simulink model "stereo_ibvs_ros_backup_20260724_144900"  (R2025b)
settings: Solver=FixedStepDiscrete  StartTime=0.0  StopTime=inf  FixedStep=cfg.Ts  RelTol=1e-3
InitFcn:
  | modelPath = get_param(bdroot,'FileName');
  |                                                                                       simulinkPath = fileparts(fileparts(modelPath));
  |                                                                                       projectRoot = fileparts(simulinkPath);
  |                                                                                       configPath = fullfile(simulinkPath,'config','stereo_ibvs_config.m');
  |                                                                                       corePath = fullfile(simulinkPath,'core');
  |                                                                                       generatedPath = fullfile(projectRoot,'matlab_msg_gen',computer('arch'),'install','m');
  |                                                                                       if ~isfile(configPath), error('StereoIBVS:ConfigNotFound','找不到配置文件：%s',configPath); end
  |                                                                                       addpath(corePath);
  |                                                                                       if isfolder(generatedPath), addpath(generatedPath,'-begin'); end
  |                                                                                       run(configPath);
undefined symbols (not defined in the file): cfg, data, data_SL_Info
libraries: ros2lib x10
settings Model: Creator=hlc  LastModifiedBy=hlc
settings DataIOCC: SaveOutput=off  SaveTime=off  ReturnWorkspaceOutputs=off

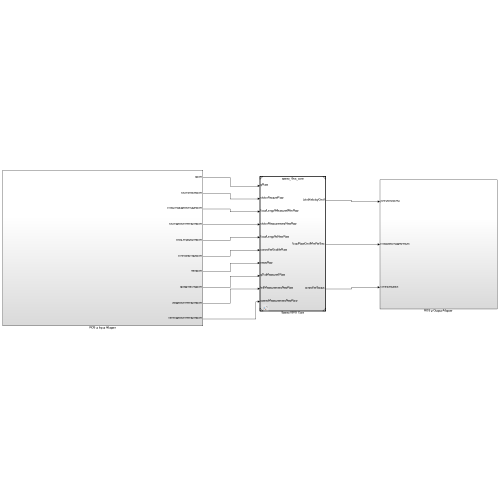
[thumbnail: Simulink's stored preview of the top-level diagram]
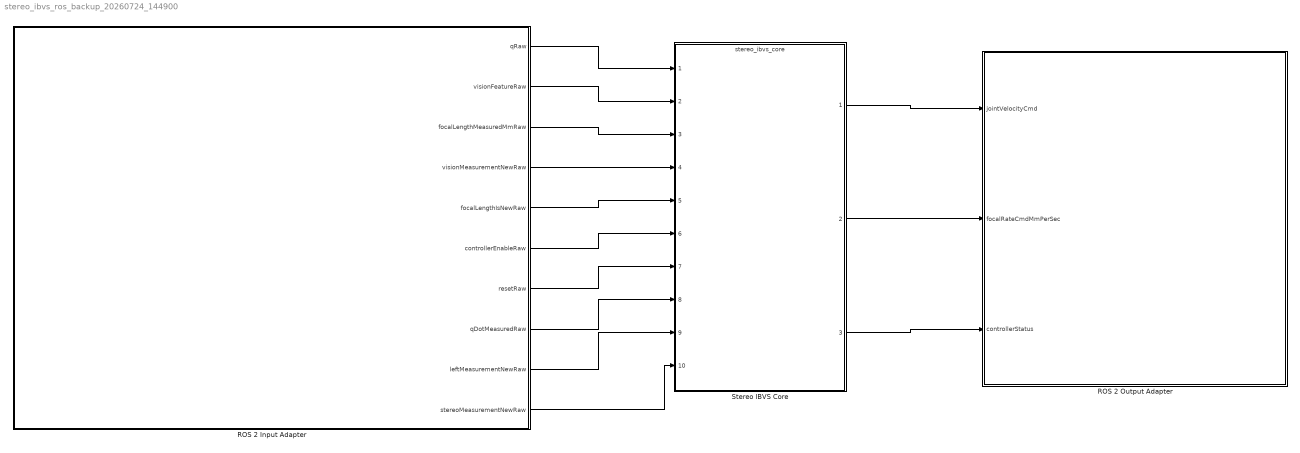
== system stereo_ibvs_ros_backup_20260724_144900 ==
  ROS 2 Input Adapter : Subsystem
  ROS 2 Output Adapter : Subsystem
  Stereo IBVS Core : ModelReference  ModelNameDialog=stereo_ibvs_core  SimulationMode=Normal  ModelReferenceVersion=1.1
  wires:
  ROS 2 Input Adapter/1(qRaw) -> Stereo IBVS Core/1
  ROS 2 Input Adapter/2(visionFeatureRaw) -> Stereo IBVS Core/2
  ROS 2 Input Adapter/3(focalLengthMeasuredMmRaw) -> Stereo IBVS Core/3
  ROS 2 Input Adapter/4(visionMeasurementNewRaw) -> Stereo IBVS Core/4
  ROS 2 Input Adapter/5(focalLengthIsNewRaw) -> Stereo IBVS Core/5
  ROS 2 Input Adapter/6(controllerEnableRaw) -> Stereo IBVS Core/6
  ROS 2 Input Adapter/7(resetRaw) -> Stereo IBVS Core/7
  ROS 2 Input Adapter/8(qDotMeasuredRaw) -> Stereo IBVS Core/8
  ROS 2 Input Adapter/9(leftMeasurementNewRaw) -> Stereo IBVS Core/9
  ROS 2 Input Adapter/10(stereoMeasurementNewRaw) -> Stereo IBVS Core/10
  Stereo IBVS Core/1 -> ROS 2 Output Adapter/1(jointVelocityCmd)
  Stereo IBVS Core/2 -> ROS 2 Output Adapter/2(focalRateCmdMmPerSec)
  Stereo IBVS Core/3 -> ROS 2 Output Adapter/3(controllerStatus)

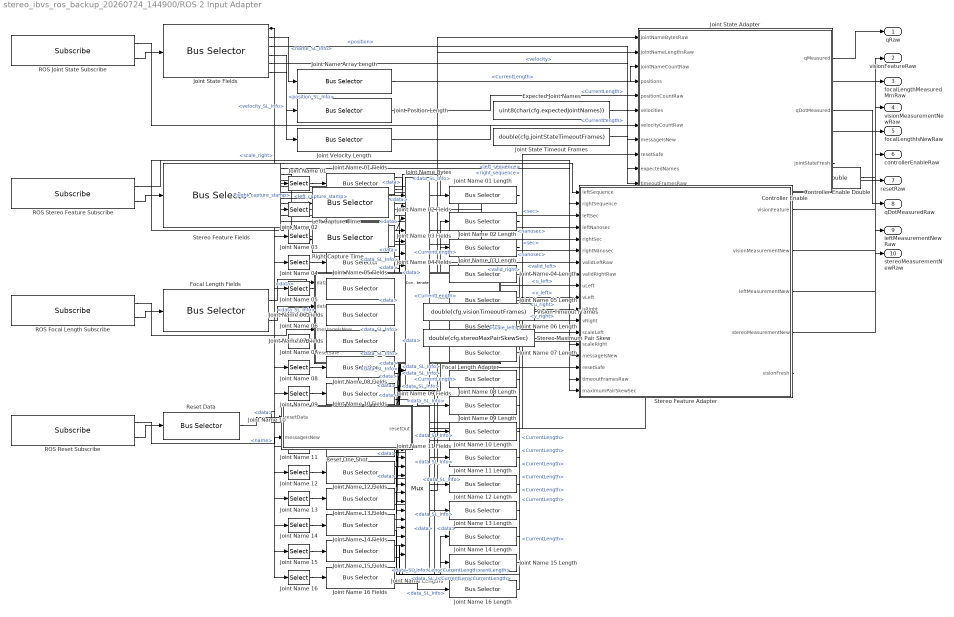
== system stereo_ibvs_ros_backup_20260724_144900/ROS 2 Input Adapter ==
  Controller Enable : Logic  AllPortsSameDT=off  OutDataTypeStr=boolean
  Controller Enable Double : DataTypeConversion  OutDataTypeStr=double  SaturateOnIntegerOverflow=off  RndMeth=Floor
  Expected Joint Names : Constant  Value=uint8(char(cfg.expectedJointNames))  SampleTime=-1
  Focal Length Adapter : MATLAB Function  TreatAsAtomicUnit=on
  Focal Length Fields : BusSelector  OutputSignals=data,data_SL_Info
  Joint Name 01 : Selector  InputPortWidth=16  IndexOptions=Index vector (dialog)  Indices=1  OutputSizes=1
  Joint Name 01 Fields : BusSelector  OutputSignals=data,data_SL_Info
  Joint Name 01 Length : BusSelector  OutputSignals=CurrentLength
  Joint Name 02 : Selector  InputPortWidth=16  IndexOptions=Index vector (dialog)  Indices=2  OutputSizes=1
  Joint Name 02 Fields : BusSelector  OutputSignals=data,data_SL_Info
  Joint Name 02 Length : BusSelector  OutputSignals=CurrentLength
  Joint Name 03 : Selector  InputPortWidth=16  IndexOptions=Index vector (dialog)  Indices=3  OutputSizes=1
  Joint Name 03 Fields : BusSelector  OutputSignals=data,data_SL_Info
  Joint Name 03 Length : BusSelector  OutputSignals=CurrentLength
  Joint Name 04 : Selector  InputPortWidth=16  IndexOptions=Index vector (dialog)  Indices=4  OutputSizes=1
  Joint Name 04 Fields : BusSelector  OutputSignals=data,data_SL_Info
  Joint Name 04 Length : BusSelector  OutputSignals=CurrentLength
  Joint Name 05 : Selector  InputPortWidth=16  IndexOptions=Index vector (dialog)  Indices=5  OutputSizes=1
  Joint Name 05 Fields : BusSelector  OutputSignals=data,data_SL_Info
  Joint Name 05 Length : BusSelector  OutputSignals=CurrentLength
  Joint Name 06 : Selector  InputPortWidth=16  IndexOptions=Index vector (dialog)  Indices=6  OutputSizes=1
  Joint Name 06 Fields : BusSelector  OutputSignals=data,data_SL_Info
  Joint Name 06 Length : BusSelector  OutputSignals=CurrentLength
  Joint Name 07 : Selector  InputPortWidth=16  IndexOptions=Index vector (dialog)  Indices=7  OutputSizes=1
  Joint Name 07 Fields : BusSelector  OutputSignals=data,data_SL_Info
  Joint Name 07 Length : BusSelector  OutputSignals=CurrentLength
  Joint Name 08 : Selector  InputPortWidth=16  IndexOptions=Index vector (dialog)  Indices=8  OutputSizes=1
  Joint Name 08 Fields : BusSelector  OutputSignals=data,data_SL_Info
  Joint Name 08 Length : BusSelector  OutputSignals=CurrentLength
  Joint Name 09 : Selector  InputPortWidth=16  IndexOptions=Index vector (dialog)  Indices=9  OutputSizes=1
  Joint Name 09 Fields : BusSelector  OutputSignals=data,data_SL_Info
  Joint Name 09 Length : BusSelector  OutputSignals=CurrentLength
  Joint Name 10 : Selector  InputPortWidth=16  IndexOptions=Index vector (dialog)  Indices=10  OutputSizes=1
  Joint Name 10 Fields : BusSelector  OutputSignals=data,data_SL_Info
  Joint Name 10 Length : BusSelector  OutputSignals=CurrentLength
  Joint Name 11 : Selector  InputPortWidth=16  IndexOptions=Index vector (dialog)  Indices=11  OutputSizes=1
  Joint Name 11 Fields : BusSelector  OutputSignals=data,data_SL_Info
  Joint Name 11 Length : BusSelector  OutputSignals=CurrentLength
  Joint Name 12 : Selector  InputPortWidth=16  IndexOptions=Index vector (dialog)  Indices=12  OutputSizes=1
  Joint Name 12 Fields : BusSelector  OutputSignals=data,data_SL_Info
  Joint Name 12 Length : BusSelector  OutputSignals=CurrentLength
  Joint Name 13 : Selector  InputPortWidth=16  IndexOptions=Index vector (dialog)  Indices=13  OutputSizes=1
  Joint Name 13 Fields : BusSelector  OutputSignals=data,data_SL_Info
  Joint Name 13 Length : BusSelector  OutputSignals=CurrentLength
  Joint Name 14 : Selector  InputPortWidth=16  IndexOptions=Index vector (dialog)  Indices=14  OutputSizes=1
  Joint Name 14 Fields : BusSelector  OutputSignals=data,data_SL_Info
  Joint Name 14 Length : BusSelector  OutputSignals=CurrentLength
  Joint Name 15 : Selector  InputPortWidth=16  IndexOptions=Index vector (dialog)  Indices=15  OutputSizes=1
  Joint Name 15 Fields : BusSelector  OutputSignals=data,data_SL_Info
  Joint Name 15 Length : BusSelector  OutputSignals=CurrentLength
  Joint Name 16 : Selector  InputPortWidth=16  IndexOptions=Index vector (dialog)  Indices=16  OutputSizes=1
  Joint Name 16 Fields : BusSelector  OutputSignals=data,data_SL_Info
  Joint Name 16 Length : BusSelector  OutputSignals=CurrentLength
  Joint Name Array Length : BusSelector  OutputSignals=CurrentLength
  Joint Name Bytes : Concatenate  NumInputs=16
  Joint Name Lengths : Mux  Inputs=16
  Joint Position Length : BusSelector  OutputSignals=CurrentLength
  Joint State Adapter : MATLAB Function  TreatAsAtomicUnit=on
  Joint State Fields : BusSelector  OutputSignals=name,name_SL_Info,position,position_SL_Info,velocity,velocity_SL_Info
  Joint State Timeout Frames : Constant  Value=double(cfg.jointStateTimeoutFrames)  OutDataTypeStr=double  SampleTime=-1
  Joint Velocity Length : BusSelector  OutputSignals=CurrentLength
  Left Capture Time : BusSelector  OutputSignals=sec,nanosec
  ROS Focal Length Subscribe : ros2lib/Subscribe  topicSource=Specify your own  topic=/stereo/focal_length  messageType=std_msgs/Float64MultiArray  sampleTime=cfg.Ts  QOSHistory=Keep last  QOSDepth=10  QOSReliability=Reliable  QOSDurability=Volatile  QOSDeadline=Inf  QOSLifespan=Inf  QOSLiveliness=Automatic  QOSLeaseDuration=Inf  QOSAvoidROSNamespaceConventions=off
  ROS Joint State Subscribe : ros2lib/Subscribe  topicSource=Specify your own  topic=/franka/joint_states  messageType=sensor_msgs/JointState  sampleTime=cfg.Ts  QOSHistory=Keep last  QOSDepth=10  QOSReliability=Reliable  QOSDurability=Volatile  QOSDeadline=Inf  QOSLifespan=Inf  QOSLiveliness=Automatic  QOSLeaseDuration=Inf  QOSAvoidROSNamespaceConventions=off
  ROS Reset Subscribe : ros2lib/Subscribe  topicSource=Specify your own  topic=/simulink/reset  messageType=std_msgs/Bool  sampleTime=cfg.Ts  QOSHistory=Keep last  QOSDepth=10  QOSReliability=Reliable  QOSDurability=Volatile  QOSDeadline=Inf  QOSLifespan=Inf  QOSLiveliness=Automatic  QOSLeaseDuration=Inf  QOSAvoidROSNamespaceConventions=off
  ROS Stereo Feature Subscribe : ros2lib/Subscribe  topicSource=Specify your own  topic=/vision_double/stereo_features  messageType=velocity_servo_tag_interfaces/StereoFeatures  sampleTime=cfg.Ts  QOSHistory=Keep last  QOSDepth=10  QOSReliability=Reliable  QOSDurability=Volatile  QOSDeadline=Inf  QOSLifespan=Inf  QOSLiveliness=Automatic  QOSLeaseDuration=Inf  QOSAvoidROSNamespaceConventions=off
  Reset Data : BusSelector  OutputSignals=data
  Reset One Shot : MATLAB Function  TreatAsAtomicUnit=on
  Right Capture Time : BusSelector  OutputSignals=sec,nanosec
  Stereo Feature Adapter : MATLAB Function  TreatAsAtomicUnit=on
  Stereo Feature Fields : BusSelector  OutputSignals=left_sequence,right_sequence,left_capture_stamp,right_capture_stamp,valid_left,valid_right,u_left,v_left,u_right,v_right,scale_left,scale_right
  Stereo Maximum Pair Skew : Constant  Value=double(cfg.stereoMaxPairSkewSec)  OutDataTypeStr=double  SampleTime=-1
  Vision Timeout Frames : Constant  Value=double(cfg.visionTimeoutFrames)  OutDataTypeStr=double  SampleTime=-1
  qRaw : Outport  PortDimensions=[7 1]
  visionFeatureRaw : Outport  Port=2  PortDimensions=[8 1]
  focalLengthMeasuredMmRaw : Outport  Port=3  PortDimensions=[2 1]
  visionMeasurementNewRaw : Outport  Port=4  PortDimensions=1
  focalLengthIsNewRaw : Outport  Port=5  PortDimensions=1
  controllerEnableRaw : Outport  Port=6  PortDimensions=1
  resetRaw : Outport  Port=7  PortDimensions=1
  qDotMeasuredRaw : Outport  Port=8  PortDimensions=[7 1]
  leftMeasurementNewRaw : Outport  Port=9  PortDimensions=1
  stereoMeasurementNewRaw : Outport  Port=10  PortDimensions=1
  wires:
  ? -> ?
  ROS Reset Subscribe/2 -> Reset Data/1
  Reset Data/1 -> Reset One Shot/1(resetData)  "<data>"
  ROS Reset Subscribe/1 -> Reset One Shot/2(messageIsNew)
  Joint State Fields/1 -> Joint Name 01/1, Joint Name 02/1, Joint Name 03/1, Joint Name 04/1, Joint Name 05/1, Joint Name 06/1, Joint Name 07/1, Joint Name 08/1, Joint Name 09/1, Joint Name 10/1, Joint Name 11/1, Joint Name 12/1, Joint Name 13/1, Joint Name 14/1, Joint Name 15/1, Joint Name 16/1  "<name>"
  Joint Name 01/1 -> Joint Name 01 Fields/1
  Joint Name 01 Fields/1 -> Joint Name Bytes/1  "<data>"
  Joint Name 01 Fields/2 -> Joint Name 01 Length/1  "<data_SL_Info>"
  Joint Name 01 Length/1 -> Joint Name Lengths/1  "<CurrentLength>"
  Joint Name 02/1 -> Joint Name 02 Fields/1
  Joint Name 02 Fields/1 -> Joint Name Bytes/2  "<data>"
  Joint Name 02 Fields/2 -> Joint Name 02 Length/1  "<data_SL_Info>"
  Joint Name 02 Length/1 -> Joint Name Lengths/2  "<CurrentLength>"
  Joint Name 03/1 -> Joint Name 03 Fields/1
  Joint Name 03 Fields/1 -> Joint Name Bytes/3  "<data>"
  Joint Name 03 Fields/2 -> Joint Name 03 Length/1  "<data_SL_Info>"
  Joint Name 03 Length/1 -> Joint Name Lengths/3  "<CurrentLength>"
  Joint Name 04/1 -> Joint Name 04 Fields/1
  Joint Name 04 Fields/1 -> Joint Name Bytes/4  "<data>"
  Joint Name 04 Fields/2 -> Joint Name 04 Length/1  "<data_SL_Info>"
  Joint Name 04 Length/1 -> Joint Name Lengths/4  "<CurrentLength>"
  Joint Name 05/1 -> Joint Name 05 Fields/1
  Joint Name 05 Fields/1 -> Joint Name Bytes/5  "<data>"
  Joint Name 05 Fields/2 -> Joint Name 05 Length/1  "<data_SL_Info>"
  Joint Name 05 Length/1 -> Joint Name Lengths/5  "<CurrentLength>"
  Joint Name 06/1 -> Joint Name 06 Fields/1
  Joint Name 06 Fields/1 -> Joint Name Bytes/6  "<data>"
  Joint Name 06 Fields/2 -> Joint Name 06 Length/1  "<data_SL_Info>"
  Joint Name 06 Length/1 -> Joint Name Lengths/6  "<CurrentLength>"
  Joint Name 07/1 -> Joint Name 07 Fields/1
  Joint Name 07 Fields/1 -> Joint Name Bytes/7  "<data>"
  Joint Name 07 Fields/2 -> Joint Name 07 Length/1  "<data_SL_Info>"
  Joint Name 07 Length/1 -> Joint Name Lengths/7  "<CurrentLength>"
  Joint Name 08/1 -> Joint Name 08 Fields/1
  Joint Name 08 Fields/1 -> Joint Name Bytes/8  "<data>"
  Joint Name 08 Fields/2 -> Joint Name 08 Length/1  "<data_SL_Info>"
  Joint Name 08 Length/1 -> Joint Name Lengths/8  "<CurrentLength>"
  Joint Name 09/1 -> Joint Name 09 Fields/1
  Joint Name 09 Fields/1 -> Joint Name Bytes/9  "<data>"
  Joint Name 09 Fields/2 -> Joint Name 09 Length/1  "<data_SL_Info>"
  Joint Name 09 Length/1 -> Joint Name Lengths/9  "<CurrentLength>"
  Joint Name 10/1 -> Joint Name 10 Fields/1
  Joint Name 10 Fields/1 -> Joint Name Bytes/10  "<data>"
  Joint Name 10 Fields/2 -> Joint Name 10 Length/1  "<data_SL_Info>"
  Joint Name 10 Length/1 -> Joint Name Lengths/10  "<CurrentLength>"
  Joint Name 11/1 -> Joint Name 11 Fields/1
  Joint Name 11 Fields/1 -> Joint Name Bytes/11  "<data>"
  Joint Name 11 Fields/2 -> Joint Name 11 Length/1  "<data_SL_Info>"
  Joint Name 11 Length/1 -> Joint Name Lengths/11  "<CurrentLength>"
  Joint Name 12/1 -> Joint Name 12 Fields/1
  Joint Name 12 Fields/1 -> Joint Name Bytes/12  "<data>"
  Joint Name 12 Fields/2 -> Joint Name 12 Length/1  "<data_SL_Info>"
  Joint Name 12 Length/1 -> Joint Name Lengths/12  "<CurrentLength>"
  Joint Name 13/1 -> Joint Name 13 Fields/1
  Joint Name 13 Fields/1 -> Joint Name Bytes/13  "<data>"
  Joint Name 13 Fields/2 -> Joint Name 13 Length/1  "<data_SL_Info>"
  Joint Name 13 Length/1 -> Joint Name Lengths/13  "<CurrentLength>"
  Joint Name 14/1 -> Joint Name 14 Fields/1
  Joint Name 14 Fields/1 -> Joint Name Bytes/14  "<data>"
  Joint Name 14 Fields/2 -> Joint Name 14 Length/1  "<data_SL_Info>"
  Joint Name 14 Length/1 -> Joint Name Lengths/14  "<CurrentLength>"
  Joint Name 15/1 -> Joint Name 15 Fields/1
  Joint Name 15 Fields/1 -> Joint Name Bytes/15  "<data>"
  Joint Name 15 Fields/2 -> Joint Name 15 Length/1  "<data_SL_Info>"
  Joint Name 15 Length/1 -> Joint Name Lengths/15  "<CurrentLength>"
  Joint Name 16/1 -> Joint Name 16 Fields/1
  Joint Name 16 Fields/1 -> Joint Name Bytes/16  "<data>"
  Joint Name 16 Fields/2 -> Joint Name 16 Length/1  "<data_SL_Info>"
  Joint Name 16 Length/1 -> Joint Name Lengths/16  "<CurrentLength>"
  ROS Joint State Subscribe/2 -> Joint State Fields/1
  Joint State Fields/2 -> Joint Name Array Length/1  "<name_SL_Info>"
  Joint State Fields/4 -> Joint Position Length/1  "<position_SL_Info>"
  Joint State Fields/6 -> Joint Velocity Length/1  "<velocity_SL_Info>"
  Joint Name Bytes/1 -> Joint State Adapter/1(jointNameBytesRaw)
  Joint Name Lengths/1 -> Joint State Adapter/2(jointNameLengthsRaw)
  Joint Name Array Length/1 -> Joint State Adapter/3(jointNameCountRaw)  "<CurrentLength>"
  Joint State Fields/3 -> Joint State Adapter/4(positions)  "<position>"
  Joint Position Length/1 -> Joint State Adapter/5(positionCountRaw)  "<CurrentLength>"
  Joint State Fields/5 -> Joint State Adapter/6(velocities)  "<velocity>"
  Joint Velocity Length/1 -> Joint State Adapter/7(velocityCountRaw)  "<CurrentLength>"
  ROS Joint State Subscribe/1 -> Joint State Adapter/8(messageIsNew)
  Reset One Shot/1(resetOut) -> Joint State Adapter/9(resetSafe), Stereo Feature Adapter/16(resetSafe), Focal Length Adapter/4(resetSafe), resetRaw/1
  Expected Joint Names/1 -> Joint State Adapter/10(expectedNames)
  Joint State Timeout Frames/1 -> Joint State Adapter/11(timeoutFramesRaw)
  ROS Stereo Feature Subscribe/2 -> Stereo Feature Fields/1
  Stereo Feature Fields/3 -> Left Capture Time/1  "<left_capture_stamp>"
  Stereo Feature Fields/4 -> Right Capture Time/1  "<right_capture_stamp>"
  Stereo Feature Fields/1 -> Stereo Feature Adapter/1(leftSequence)  "<left_sequence>"
  Stereo Feature Fields/2 -> Stereo Feature Adapter/2(rightSequence)  "<right_sequence>"
  Left Capture Time/1 -> Stereo Feature Adapter/3(leftSec)  "<sec>"
  Left Capture Time/2 -> Stereo Feature Adapter/4(leftNanosec)  "<nanosec>"
  Right Capture Time/1 -> Stereo Feature Adapter/5(rightSec)  "<sec>"
  Right Capture Time/2 -> Stereo Feature Adapter/6(rightNanosec)  "<nanosec>"
  Stereo Feature Fields/5 -> Stereo Feature Adapter/7(validLeftRaw)  "<valid_left>"
  Stereo Feature Fields/6 -> Stereo Feature Adapter/8(validRightRaw)  "<valid_right>"
  Stereo Feature Fields/7 -> Stereo Feature Adapter/9(uLeft)  "<u_left>"
  Stereo Feature Fields/8 -> Stereo Feature Adapter/10(vLeft)  "<v_left>"
  Stereo Feature Fields/9 -> Stereo Feature Adapter/11(uRight)  "<u_right>"
  Stereo Feature Fields/10 -> Stereo Feature Adapter/12(vRight)  "<v_right>"
  Stereo Feature Fields/11 -> Stereo Feature Adapter/13(scaleLeft)  "<scale_left>"
  Stereo Feature Fields/12 -> Stereo Feature Adapter/14(scaleRight)  "<scale_right>"
  ROS Stereo Feature Subscribe/1 -> Stereo Feature Adapter/15(messageIsNew)
  Vision Timeout Frames/1 -> Stereo Feature Adapter/17(timeoutFramesRaw)
  Stereo Maximum Pair Skew/1 -> Stereo Feature Adapter/18(maximumPairSkewSec)
  ROS Focal Length Subscribe/2 -> Focal Length Fields/1
  Focal Length Fields/1 -> Focal Length Adapter/1(data)  "<data>"
  Focal Length Fields/2 -> Focal Length Adapter/2(dataInfo)  "<data_SL_Info>"
  ROS Focal Length Subscribe/1 -> Focal Length Adapter/3(messageIsNew)
  Joint State Adapter/3(jointStateFresh) -> Controller Enable/1
  Stereo Feature Adapter/5(visionFresh) -> Controller Enable/2
  Controller Enable/1 -> Controller Enable Double/1
  Joint State Adapter/1(qMeasured) -> qRaw/1
  Stereo Feature Adapter/1(visionFeature) -> visionFeatureRaw/1
  Focal Length Adapter/1(focalLengthMeasuredMm) -> focalLengthMeasuredMmRaw/1
  Stereo Feature Adapter/2(visionMeasurementNew) -> visionMeasurementNewRaw/1
  Focal Length Adapter/2(focalLengthIsNew) -> focalLengthIsNewRaw/1
  Controller Enable Double/1 -> controllerEnableRaw/1
  Joint State Adapter/2(qDotMeasured) -> qDotMeasuredRaw/1
  Stereo Feature Adapter/3(leftMeasurementNew) -> leftMeasurementNewRaw/1
  Stereo Feature Adapter/4(stereoMeasurementNew) -> stereoMeasurementNewRaw/1

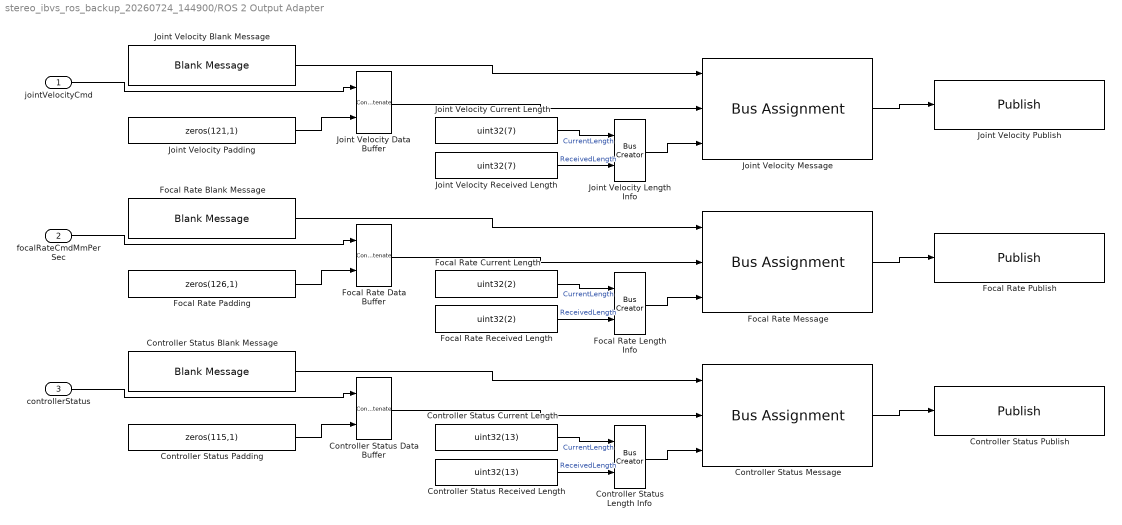
== system stereo_ibvs_ros_backup_20260724_144900/ROS 2 Output Adapter ==
  jointVelocityCmd : Inport  PortDimensions=[7 1]
  focalRateCmdMmPerSec : Inport  Port=2  PortDimensions=[2 1]
  controllerStatus : Inport  Port=3  PortDimensions=[13 1]
  Controller Status Blank Message : ros2lib/Blank Message  messageClass=Message  entityType=std_msgs/Float64MultiArray  messageType=std_msgs/Float64MultiArray  SampleTime=cfg.Ts
  Controller Status Current Length : Constant  Value=uint32(13)  OutDataTypeStr=uint32  SampleTime=-1
  Controller Status Data Buffer : Concatenate
  Controller Status Length Info : BusCreator  Inputs=2  OutDataTypeStr=Bus: SL_Bus_ROSVariableLengthArrayInfo
  Controller Status Message : BusAssignment  AssignedSignals=data,data_SL_Info
  Controller Status Padding : Constant  Value=zeros(115,1)  OutDataTypeStr=double  SampleTime=-1
  Controller Status Publish : ros2lib/Publish  topicSource=Specify your own  topic=/simulink/controller_status  messageType=std_msgs/Float64MultiArray  QOSHistory=Keep last  QOSDepth=10  QOSReliability=Reliable  QOSDurability=Volatile  QOSDeadline=Inf  QOSLifespan=Inf  QOSLiveliness=Automatic  QOSLeaseDuration=Inf  QOSAvoidROSNamespaceConventions=off
  Controller Status Received Length : Constant  Value=uint32(13)  OutDataTypeStr=uint32  SampleTime=-1
  Focal Rate Blank Message : ros2lib/Blank Message  messageClass=Message  entityType=std_msgs/Float64MultiArray  messageType=std_msgs/Float64MultiArray  SampleTime=cfg.Ts
  Focal Rate Current Length : Constant  Value=uint32(2)  OutDataTypeStr=uint32  SampleTime=-1
  Focal Rate Data Buffer : Concatenate
  Focal Rate Length Info : BusCreator  Inputs=2  OutDataTypeStr=Bus: SL_Bus_ROSVariableLengthArrayInfo
  Focal Rate Message : BusAssignment  AssignedSignals=data,data_SL_Info
  Focal Rate Padding : Constant  Value=zeros(126,1)  OutDataTypeStr=double  SampleTime=-1
  Focal Rate Publish : ros2lib/Publish  topicSource=Specify your own  topic=/simulink/focal_rate_cmd  messageType=std_msgs/Float64MultiArray  QOSHistory=Keep last  QOSDepth=10  QOSReliability=Reliable  QOSDurability=Volatile  QOSDeadline=Inf  QOSLifespan=Inf  QOSLiveliness=Automatic  QOSLeaseDuration=Inf  QOSAvoidROSNamespaceConventions=off
  Focal Rate Received Length : Constant  Value=uint32(2)  OutDataTypeStr=uint32  SampleTime=-1
  Joint Velocity Blank Message : ros2lib/Blank Message  messageClass=Message  entityType=std_msgs/Float64MultiArray  messageType=std_msgs/Float64MultiArray  SampleTime=cfg.Ts
  Joint Velocity Current Length : Constant  Value=uint32(7)  OutDataTypeStr=uint32  SampleTime=-1
  Joint Velocity Data Buffer : Concatenate
  Joint Velocity Length Info : BusCreator  Inputs=2  OutDataTypeStr=Bus: SL_Bus_ROSVariableLengthArrayInfo
  Joint Velocity Message : BusAssignment  AssignedSignals=data,data_SL_Info
  Joint Velocity Padding : Constant  Value=zeros(121,1)  OutDataTypeStr=double  SampleTime=-1
  Joint Velocity Publish : ros2lib/Publish  topicSource=Specify your own  topic=/simulink/target_joints_velocities  messageType=std_msgs/Float64MultiArray  QOSHistory=Keep last  QOSDepth=10  QOSReliability=Reliable  QOSDurability=Volatile  QOSDeadline=Inf  QOSLifespan=Inf  QOSLiveliness=Automatic  QOSLeaseDuration=Inf  QOSAvoidROSNamespaceConventions=off
  Joint Velocity Received Length : Constant  Value=uint32(7)  OutDataTypeStr=uint32  SampleTime=-1
  wires:
  ? -> ?
  jointVelocityCmd/1 -> Joint Velocity Data Buffer/1
  Joint Velocity Padding/1 -> Joint Velocity Data Buffer/2
  Joint Velocity Current Length/1 -> Joint Velocity Length Info/1  "CurrentLength"
  Joint Velocity Received Length/1 -> Joint Velocity Length Info/2  "ReceivedLength"
  Joint Velocity Blank Message/1 -> Joint Velocity Message/1
  Joint Velocity Data Buffer/1 -> Joint Velocity Message/2
  Joint Velocity Length Info/1 -> Joint Velocity Message/3
  Joint Velocity Message/1 -> Joint Velocity Publish/1
  focalRateCmdMmPerSec/1 -> Focal Rate Data Buffer/1
  Focal Rate Padding/1 -> Focal Rate Data Buffer/2
  Focal Rate Current Length/1 -> Focal Rate Length Info/1  "CurrentLength"
  Focal Rate Received Length/1 -> Focal Rate Length Info/2  "ReceivedLength"
  Focal Rate Blank Message/1 -> Focal Rate Message/1
  Focal Rate Data Buffer/1 -> Focal Rate Message/2
  Focal Rate Length Info/1 -> Focal Rate Message/3
  Focal Rate Message/1 -> Focal Rate Publish/1
  controllerStatus/1 -> Controller Status Data Buffer/1
  Controller Status Padding/1 -> Controller Status Data Buffer/2
  Controller Status Current Length/1 -> Controller Status Length Info/1  "CurrentLength"
  Controller Status Received Length/1 -> Controller Status Length Info/2  "ReceivedLength"
  Controller Status Blank Message/1 -> Controller Status Message/1
  Controller Status Data Buffer/1 -> Controller Status Message/2
  Controller Status Length Info/1 -> Controller Status Message/3
  Controller Status Message/1 -> Controller Status Publish/1

== matlab function stereo_ibvs_ros_backup_20260724_144900/ROS 2 Input Adapter/Joint State Adapter ==
  data: jointNameBytesRaw input; qMeasured output; jointNameLengthsRaw input; jointNameCountRaw input; positions input; positionCountRaw input; velocities input; velocityCountRaw input; messageIsNew input; resetSafe input; expectedNames input; timeoutFramesRaw input; qDotMeasured output; jointStateFresh output
function [qMeasured,qDotMeasured,jointStateFresh] = fcn( ...
    jointNameBytesRaw, ...
    jointNameLengthsRaw, ...
    jointNameCountRaw, ...
    positions, ...
    positionCountRaw, ...
    velocities, ...
    velocityCountRaw, ...
    messageIsNew, ...
    resetSafe, ...
    expectedNames, ...
    timeoutFramesRaw)
%#codegen
% 本函数按JointState.name重排七个关节的位置和实测速度，并监控反馈超时。

persistent lastQ
persistent lastQDot
persistent receivedOnce
persistent framesSinceLastValidMessage

timeoutFrames = max(1.0,floor(timeoutFramesRaw));

if isempty(lastQ)
    lastQ = zeros(7,1);
    lastQDot = zeros(7,1);
    receivedOnce = false;
    framesSinceLastValidMessage = timeoutFrames;
end

if isfinite(resetSafe) && resetSafe > 0.5
    lastQ = zeros(7,1);
    lastQDot = zeros(7,1);
    receivedOnce = false;
    framesSinceLastValidMessage = timeoutFrames;
end

newValidMessage = false;

if isfinite(messageIsNew) && messageIsNew > 0.5
    jointNameBytes = reshape(jointNameBytesRaw,128,16);
    jointNameLengths = reshape(jointNameLengthsRaw,16,1);
    nameCount = min(double(jointNameCountRaw),16.0);
    positionCount = min(double(positionCountRaw),double(numel(positions)));
    velocityCount = min(double(velocityCountRaw),double(numel(velocities)));
    sourceCount = floor(min(nameCount,min(positionCount,velocityCount)));
    expectedNameLength = size(expectedNames,2);

    candidateQ = zeros(7,1);
    candidateQDot = zeros(7,1);
    found = false(7,1);

    for sourceIndex = 1:sourceCount
        sourceNameLength = double(jointNameLengths(sourceIndex));

        if sourceNameLength == expectedNameLength
            sourceName = jointNameBytes(1:expectedNameLength,sourceIndex);

            for targetIndex = 1:7
                expectedName = expectedNames(targetIndex,:).';

                if all(sourceName == expectedName)
                    if ~found(targetIndex)
                        candidateQ(targetIndex) = positions(sourceIndex);
                        candidateQDot(targetIndex) = velocities(sourceIndex);
                        found(targetIndex) = true;
                    end
                end
            end
        end
    end

    newValidMessage = ...
        all(found) && ...
        all(isfinite(candidateQ)) && ...
        all(isfinite(candidateQDot));

    if newValidMessage
        lastQ = candidateQ;
        lastQDot = candidateQDot;
        receivedOnce = true;
        framesSinceLastValidMessage = 0;
    end
end

if ~newValidMessage && receivedOnce
    framesSinceLastValidMessage = min( ...
        framesSinceLastValidMessage + 1, ...
        timeoutFrames + 1);
end

qMeasured = lastQ;
qDotMeasured = lastQDot;
jointStateFresh = double( ...
    receivedOnce && ...
    framesSinceLastValidMessage < timeoutFrames);
end

== matlab function stereo_ibvs_ros_backup_20260724_144900/ROS 2 Input Adapter/Reset One Shot ==
  data: resetData input; resetOut output; messageIsNew input
function resetOut = fcn(resetData,messageIsNew)
%#codegen
% 本函数仅在收到一条新的 true 消息时输出单周期复位脉冲。
resetOut = double( ...
    isfinite(double(resetData)) && ...
    isfinite(messageIsNew) && ...
    logical(resetData) && ...
    messageIsNew > 0.5);
end

== matlab function stereo_ibvs_ros_backup_20260724_144900/ROS 2 Input Adapter/Stereo Feature Adapter ==
  data: leftSequence input; visionFeature output; rightSequence input; leftSec input; leftNanosec input; rightSec input; rightNanosec input; validLeftRaw input; validRightRaw input; uLeft input; vLeft input; uRight input; vRight input; scaleLeft input; scaleRight input; messageIsNew input; resetSafe input; timeoutFramesRaw input; maximumPairSkewSec input; visionMeasurementNew output; leftMeasurementNew output; stereoMeasurementNew output; visionFresh output
function [ ...
    visionFeature, ...
    visionMeasurementNew, ...
    leftMeasurementNew, ...
    stereoMeasurementNew, ...
    visionFresh] = fcn( ...
    leftSequence, ...
    rightSequence, ...
    leftSec, ...
    leftNanosec, ...
    rightSec, ...
    rightNanosec, ...
    validLeftRaw, ...
    validRightRaw, ...
    uLeft, ...
    vLeft, ...
    uRight, ...
    vRight, ...
    scaleLeft, ...
    scaleRight, ...
    messageIsNew, ...
    resetSafe, ...
    timeoutFramesRaw, ...
    maximumPairSkewSec)
%#codegen
% 本函数按左右帧序号识别真实新图像，并仅让新的合格双目配对触发EKF。
% 左相机可以独立刷新中心控制；右相机更新不要求左相机同步到达。

persistent lastFeature
persistent lastLeftSequence
persistent lastRightSequence
persistent pairedLeftSequence
persistent pairedRightSequence
persistent lastLeftCaptureTime
persistent lastRightCaptureTime
persistent leftSeen
persistent rightSeen
persistent stereoPairSeen
persistent framesSinceLastLeftFrame

timeoutFrames = max(1.0,floor(timeoutFramesRaw));

if isempty(lastFeature)
    lastFeature = zeros(8,1);
    lastLeftSequence = uint32(0);
    lastRightSequence = uint32(0);
    pairedLeftSequence = uint32(0);
    pairedRightSequence = uint32(0);
    lastLeftCaptureTime = 0;
    lastRightCaptureTime = 0;
    leftSeen = false;
    rightSeen = false;
    stereoPairSeen = false;
    framesSinceLastLeftFrame = timeoutFrames;
end

visionMeasurementNew = 0;
leftMeasurementNew = 0;
stereoMeasurementNew = 0;

resetRequested = ...
    isfinite(resetSafe) && ...
    resetSafe > 0.5;

if resetRequested
    lastFeature = zeros(8,1);
    lastLeftSequence = uint32(0);
    lastRightSequence = uint32(0);
    pairedLeftSequence = uint32(0);
    pairedRightSequence = uint32(0);
    lastLeftCaptureTime = 0;
    lastRightCaptureTime = 0;
    leftSeen = false;
    rightSeen = false;
    stereoPairSeen = false;
    framesSinceLastLeftFrame = timeoutFrames;
else
    leftChanged = false;
    rightChanged = false;

    if isfinite(messageIsNew) && messageIsNew > 0.5
        leftChanged = ~leftSeen || leftSequence ~= lastLeftSequence;
        rightChanged = ~rightSeen || rightSequence ~= lastRightSequence;

        leftValuesFinite = ...
            all(isfinite([double(leftSec);double(leftNanosec);uLeft;vLeft;scaleLeft]));

        rightValuesFinite = ...
            all(isfinite([double(rightSec);double(rightNanosec);uRight;vRight;scaleRight]));

        if leftChanged && leftValuesFinite
            lastLeftSequence = leftSequence;
            lastLeftCaptureTime = ...
                double(leftSec) + 1.0e-9*double(leftNanosec);
            lastFeature(1) = double(logical(validLeftRaw));
            lastFeature(3) = uLeft;
            lastFeature(4) = vLeft;
            lastFeature(7) = scaleLeft;
            leftSeen = true;
            framesSinceLastLeftFrame = 0;
            leftMeasurementNew = 1;
        else
            leftChanged = false;
        end

        if rightChanged && rightValuesFinite
            lastRightSequence = rightSequence;
            lastRightCaptureTime = ...
                double(rightSec) + 1.0e-9*double(rightNanosec);
            lastFeature(2) = double(logical(validRightRaw));
            lastFeature(5) = uRight;
            lastFeature(6) = vRight;
            lastFeature(8) = scaleRight;
            rightSeen = true;
        else
            rightChanged = false;
        end

        visionMeasurementNew = double(leftChanged || rightChanged);

        pairUnused = ...
            leftSeen && ...
            rightSeen && ...
            (~stereoPairSeen || ...
             (lastLeftSequence ~= pairedLeftSequence && ...
              lastRightSequence ~= pairedRightSequence));

        pairSkewValid = ...
            isfinite(maximumPairSkewSec) && ...
            maximumPairSkewSec >= 0 && ...
            abs(lastLeftCaptureTime-lastRightCaptureTime) <= ...
                maximumPairSkewSec;

        if pairUnused && pairSkewValid
            pairedLeftSequence = lastLeftSequence;
            pairedRightSequence = lastRightSequence;
            stereoPairSeen = true;
            stereoMeasurementNew = 1;
        end
    end

    if leftMeasurementNew < 0.5 && leftSeen
        framesSinceLastLeftFrame = min( ...
            framesSinceLastLeftFrame + 1, ...
            timeoutFrames + 1);
    end
end

visionFeature = lastFeature;
visionFresh = double( ...
    leftSeen && ...
    framesSinceLastLeftFrame < timeoutFrames);
end

== matlab function stereo_ibvs_ros_backup_20260724_144900/ROS 2 Input Adapter/Focal Length Adapter ==
  data: data input; focalLengthMeasuredMm output; dataInfo input; messageIsNew input; resetSafe input; focalLengthIsNew output
function [focalLengthMeasuredMm,focalLengthIsNew] = fcn( ...
    data, ...
    dataInfo, ...
    messageIsNew, ...
    resetSafe)
%#codegen
% 本函数读取双目焦距消息的前两个元素，并仅转发合法的新消息。

persistent lastFocalLengthMm

if isempty(lastFocalLengthMm)
    lastFocalLengthMm = zeros(2,1);
end

focalLengthIsNew = 0;

if isfinite(resetSafe) && resetSafe > 0.5
    lastFocalLengthMm = zeros(2,1);
elseif isfinite(messageIsNew) && messageIsNew > 0.5
    receivedLength = min(double(dataInfo.CurrentLength),double(numel(data)));

    if receivedLength >= 2
        candidate = reshape(data(1:2),2,1);

        if all(isfinite(candidate))
            lastFocalLengthMm = candidate;
            focalLengthIsNew = 1;
        end
    end
end

focalLengthMeasuredMm = lastFocalLengthMm;
end
